simulink model "simulateur_derniere_version"  (R2022b)
settings: Solver=ode4  StartTime=0.0  StopTime=10  FixedStep=dt  RelTol=1e-3
model workspace: external: MATLAB File /Users/antoine/Desktop/GPH/H2023/Design_2/simulation_équipe_1/init.m (data not in the file)
values from neighbouring files (symbols this model uses):
  distance_corde_capteur = 0.00382    [init.m]
  dt = 0.000125    [init.m]
  f = 110    [init.m]    (also in visualize.m = specs(3,:))
  freq_min = 80    [init.m]
  freq_min_1 = freq_min    (= 80)    [init.m]
  Longueur = 0.44    [init.m]
  mu = 0.010011363636363636    (= 0.0100113636364)    [init.m]
  n = 21    [init.m]
libraries: simulink x1, slpidlib x1, dspstat3 x1
settings Model: Creator=antoine  LastModifiedBy=antoine

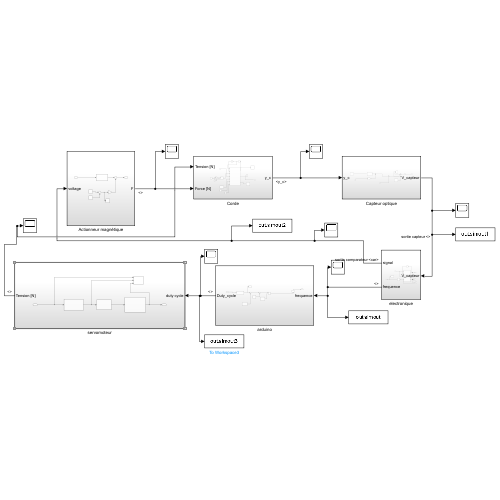
[thumbnail: Simulink's stored preview of the top-level diagram]
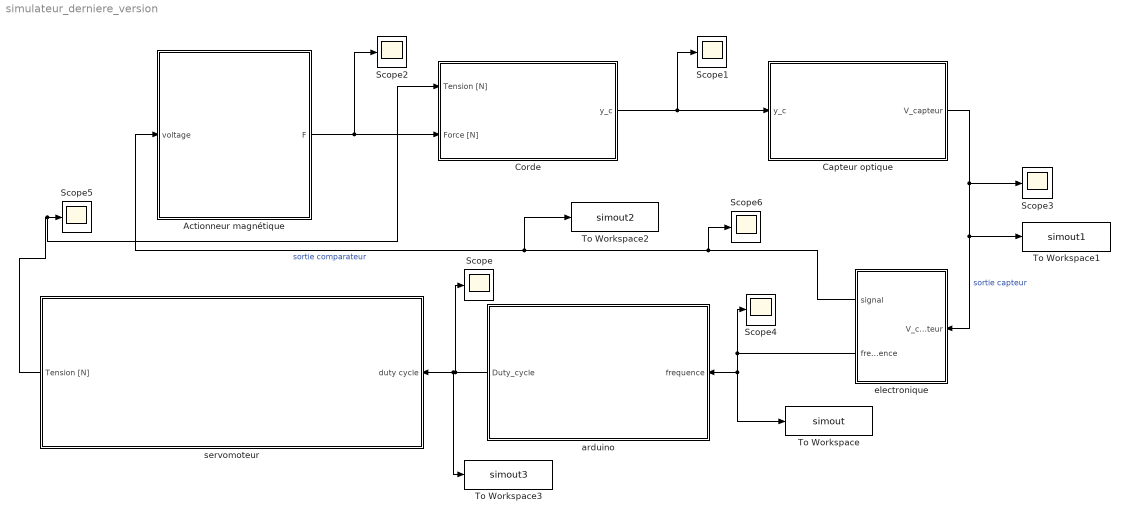
== system simulateur_derniere_version ==
  Actionneur magnétique : Subsystem
  Capteur optique : Subsystem
  Corde : Subsystem
  Scope{,1..6} (7 alike) : Scope
  To Workspace : ToWorkspace  VariableName=simout  SaveFormat=Structure  SampleTime=-1
      settings: Save2DSignal=2-D array (concatenate along first dimension)
  To Workspace1 : ToWorkspace  VariableName=simout1  SampleTime=-1
      settings: Save2DSignal=2-D array (concatenate along first dimension)
  To Workspace2 : ToWorkspace  VariableName=simout2  SampleTime=-1
      settings: Save2DSignal=2-D array (concatenate along first dimension)
  To Workspace3 : ToWorkspace  VariableName=simout3  SampleTime=-1
      settings: Save2DSignal=2-D array (concatenate along first dimension)
  arduino : Subsystem
  electronique : Subsystem
  servomoteur : Subsystem
  wires:
  Corde/1(y_c) -> Capteur optique/1(y_c), Scope1/1
  Capteur optique/1(V_capteur) -> Scope3/1, electronique/1(V_capteur), To Workspace1/1  "sortie capteur"
  servomoteur/1(Tension [N]) -> Corde/1(Tension [N]), Scope5/1
  Actionneur magnétique/1(F) -> Scope2/1, Corde/2(Force [N])
  electronique/1(signal) -> Scope6/1, To Workspace2/1, Actionneur magnétique/1(voltage)  "sortie comparateur"
  electronique/2(frequence) -> To Workspace/1, arduino/1(frequence), Scope4/1
  arduino/1(Duty_cycle) -> Scope/1, To Workspace3/1, servomoteur/1(duty cycle)

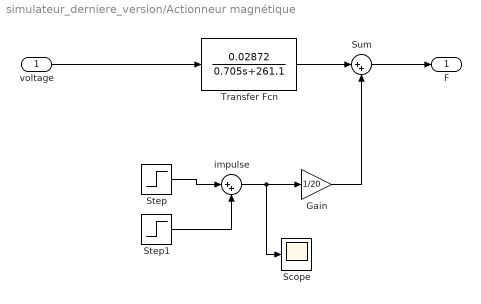
== system simulateur_derniere_version/Actionneur magnétique ==
  voltage : Inport
  Gain : Gain  Gain=1/20
  Scope : Scope
  Step : Step  Time=3*dt  SampleTime=0
  Step1 : Step  Time=6*dt  After=-1  SampleTime=0
  Sum : Sum  Inputs=|++
  Transfer Fcn : TransferFcn  Numerator=[0.02872]  Denominator=[0.705 261.1]
  impulse : Sum  Inputs=|++
  F : Outport
  wires:
  voltage/1 -> Transfer Fcn/1
  Transfer Fcn/1 -> Sum/1
  Sum/1 -> F/1
  Gain/1 -> Sum/2
  Step/1 -> impulse/1
  Step1/1 -> impulse/2
  impulse/1 -> Scope/1, Gain/1

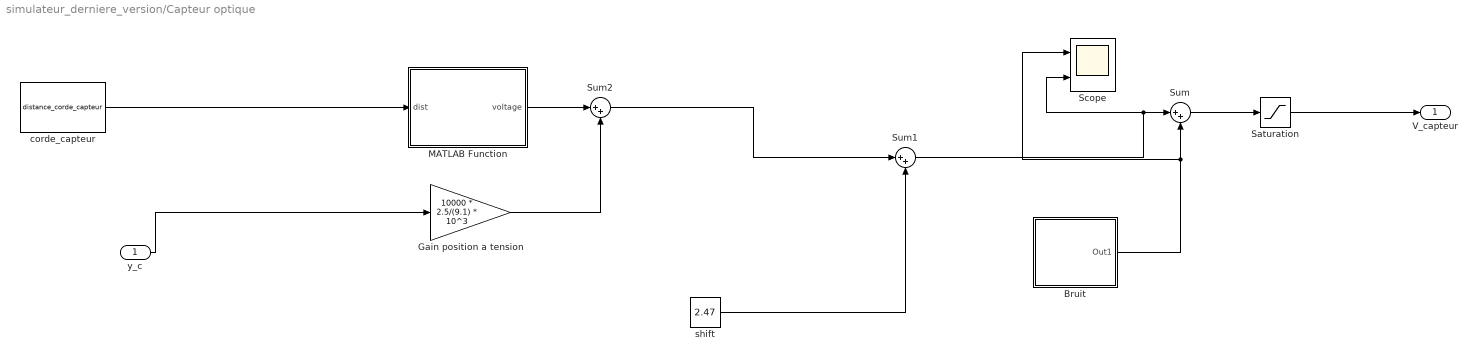
== system simulateur_derniere_version/Capteur optique ==
  y_c : Inport
  Bruit : Subsystem
  Gain position a tension : Gain  Gain=10000 * 2.5/(9.1) * 10^3
  MATLAB Function : MATLAB Function  TreatAsAtomicUnit=on
  Saturation : Saturate  UpperLimit=5  LowerLimit=0
  Scope : Scope  NumInputPorts=2
  Sum : Sum  Inputs=|++
  Sum1 : Sum  Inputs=|++
  Sum2 : Sum  Inputs=|++
  corde_capteur : Constant  Value=distance_corde_capteur
  shift : Constant  Value=2.47
  V_capteur : Outport
  wires:
  Sum/1 -> Saturation/1
  shift/1 -> Sum1/2
  Sum1/1 -> Scope/2, Sum/1
  Bruit/1(Out1) -> Scope/1, Sum/2
  Saturation/1 -> V_capteur/1
  y_c/1 -> Gain position a tension/1
  corde_capteur/1 -> MATLAB Function/1(dist)
  Gain position a tension/1 -> Sum2/2
  Sum2/1 -> Sum1/1
  MATLAB Function/1(voltage) -> Sum2/1

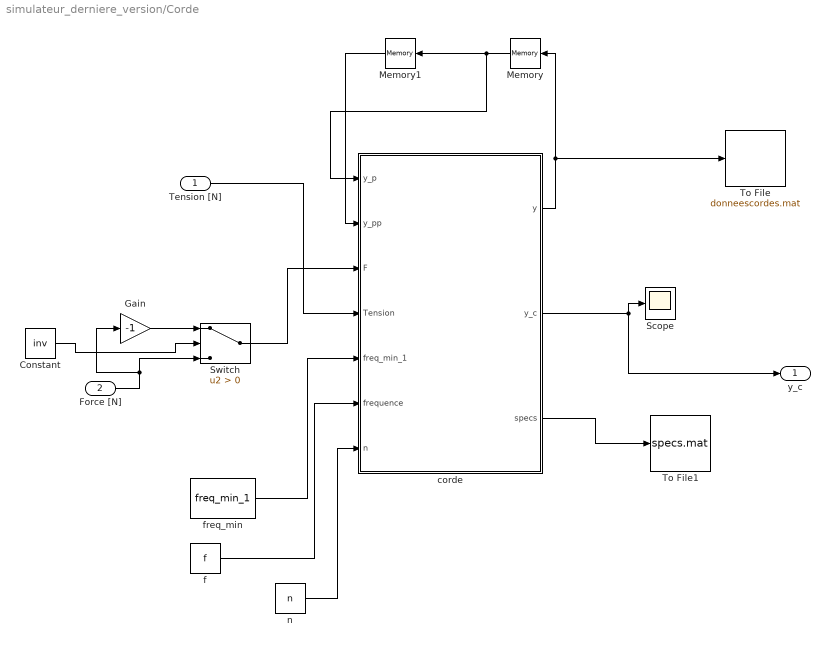
== system simulateur_derniere_version/Corde ==
  Tension [N] : Inport
  Force [N] : Inport  Port=2
  Constant : Constant  Value=inv
  Gain : Gain  Gain=-1
  Memory : Memory
  Memory1 : Memory
  Scope : Scope
  Switch : Switch  Criteria=u2 > Threshold  SaturateOnIntegerOverflow=off  InputSameDT=off
  To File : ToFile  Filename=donneescordes.mat  SaveFormat=Timeseries
  To File1 : ToFile  Filename=specs.mat  MatrixName=specs
  corde : MATLAB Function  TreatAsAtomicUnit=on
  f : Constant  Value=f
  freq_min : Constant  Value=freq_min_1
  n : Constant  Value=n
  y_c : Outport
  wires:
  corde/2(y_c) -> y_c/1, Scope/1
  Memory/1 -> corde/1(y_p), Memory1/1
  Memory1/1 -> corde/2(y_pp)
  corde/1(y) -> Memory/1, To File/1
  Switch/1 -> corde/3(F)
  Gain/1 -> Switch/1
  Force [N]/1 -> Switch/3, Gain/1
  Constant/1 -> Switch/2
  Tension [N]/1 -> corde/4(Tension)
  corde/3(specs) -> To File1/1
  freq_min/1 -> corde/5(freq_min_1)
  f/1 -> corde/6(frequence)
  n/1 -> corde/7(n)

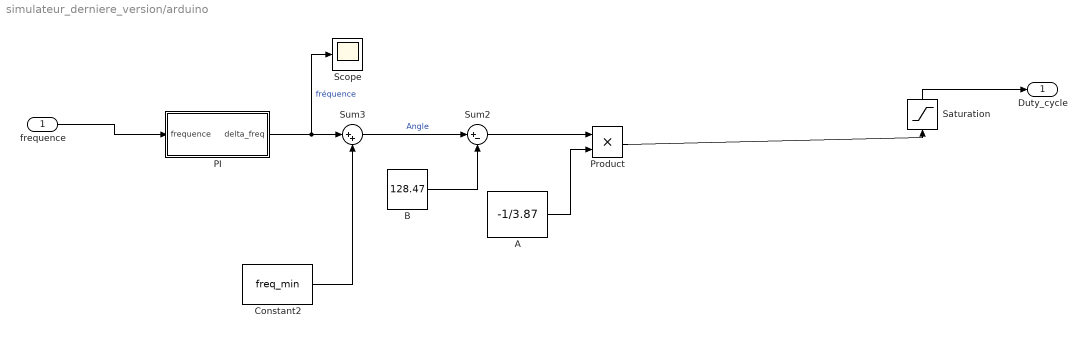
== system simulateur_derniere_version/arduino ==
  frequence : Inport
  A : Constant  Value=-1/3.87
  B : Constant  Value=128.47
  Constant2 : Constant  Value=freq_min
  PI : Subsystem
  Product : Product
  Saturation : Saturate  UpperLimit=11.79  LowerLimit=2.72
  Scope : Scope
  Sum2 : Sum  Inputs=|+-
  Sum3 : Sum  Inputs=|++
  Duty_cycle : Outport
  wires:
  PI/1(delta_freq) -> Sum3/1, Scope/1  "fréquence"
  frequence/1 -> PI/1(frequence)
  Saturation/1 -> Duty_cycle/1
  B/1 -> Sum2/2
  Sum2/1 -> Product/1
  A/1 -> Product/2
  Product/1 -> Saturation/1
  Sum3/1 -> Sum2/1  "Angle"
  Constant2/1 -> Sum3/2

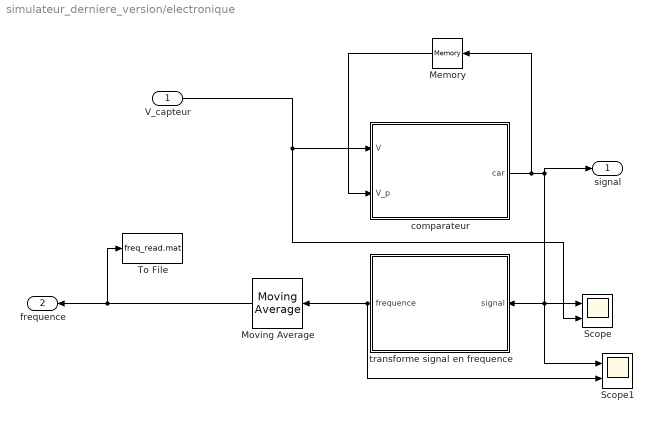
== system simulateur_derniere_version/electronique ==
  V_capteur : Inport
  Memory : Memory
  Moving Average : dspstat3/Moving Average  Method=Sliding window  ForgettingFactorPort=off  SpecifyWindowLength=on  WindowLength=100  OverlapLength=99  AllowArbitraryInputLength=off  ForgettingFactor=0.99  SimulateUsing=Interpreted execution
  Scope : Scope  NumInputPorts=2
  Scope1 : Scope  NumInputPorts=2
  To File : ToFile  Filename=freq_read.mat  MatrixName=freq
  comparateur : MATLAB Function  TreatAsAtomicUnit=on
  transforme signal en frequence : Subsystem
  signal : Outport
  frequence : Outport  Port=2
  wires:
  comparateur/1(car) -> Scope1/1, transforme signal en frequence/1(signal), Scope/1, signal/1, Memory/1
  Memory/1 -> comparateur/2(V_p)
  V_capteur/1 -> Scope/2, comparateur/1(V)
  transforme signal en frequence/1(frequence) -> Scope1/2, Moving Average/1
  Moving Average/1 -> To File/1, frequence/1

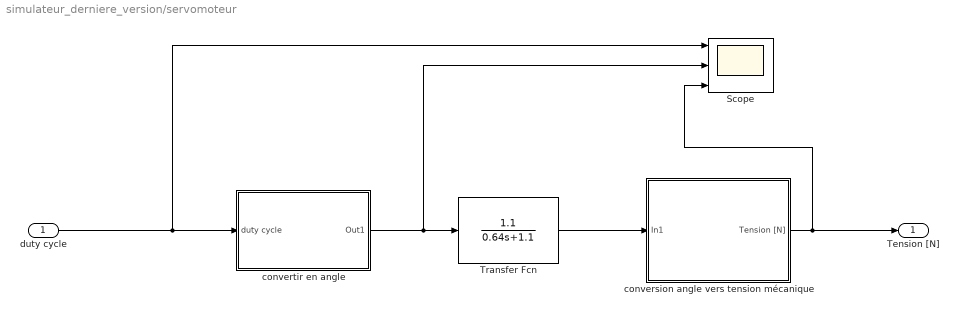
== system simulateur_derniere_version/servomoteur ==
  duty cycle : Inport
  Scope : Scope  NumInputPorts=3
  Transfer Fcn : TransferFcn  Numerator=[1.1]  Denominator=[0.64 1.1]
  conversion angle vers tension mécanique : Subsystem
  convertir en angle : Subsystem
  Tension [N] : Outport
  wires:
  convertir en angle/1(Out1) -> Transfer Fcn/1, Scope/2
  conversion angle vers tension mécanique/1(Tension [N]) -> Scope/3, Tension [N]/1
  duty cycle/1 -> Scope/1, convertir en angle/1(duty cycle)
  Transfer Fcn/1 -> conversion angle vers tension mécanique/1(In1)

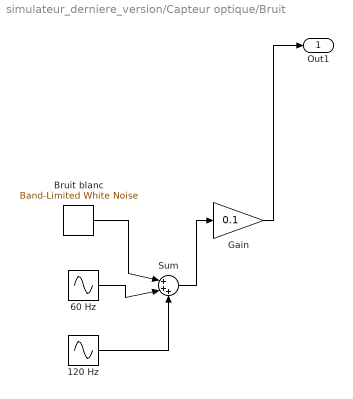
== system simulateur_derniere_version/Capteur optique/Bruit ==
  120 Hz : Sin  Frequency=120  SampleTime=0
  60 Hz : Sin  Frequency=60  SampleTime=0
  Bruit blanc : simulink/Sources/Band-Limited White Noise  Cov=[0.1]  Ts=0.1  seed=[23341]
  Gain : Gain  Gain=0.1
  Sum : Sum  Inputs=|+++
  Out1 : Outport
  wires:
  Bruit blanc/1 -> Sum/1
  60 Hz/1 -> Sum/2
  120 Hz/1 -> Sum/3
  Sum/1 -> Gain/1
  Gain/1 -> Out1/1

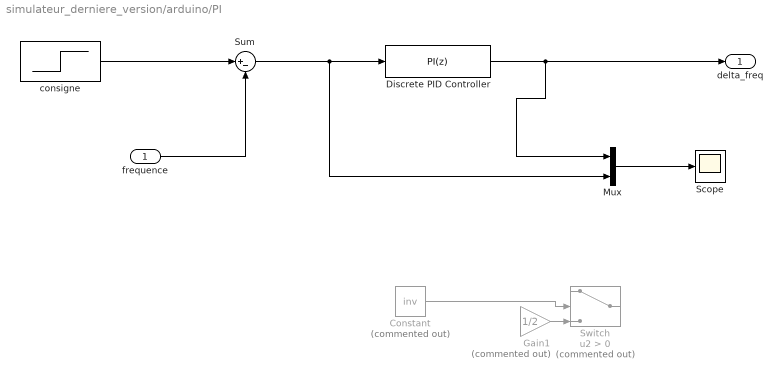
== system simulateur_derniere_version/arduino/PI ==
  frequence : Inport
  Constant : Constant  Commented=on  Value=inv
  Discrete PID Controller : slpidlib/PID Controller  Controller=PI  Form=Ideal  TimeDomain=Discrete-time  UseExternalTs=off  SampleTime=-1  IntegratorMethod=Trapezoidal  FilterMethod=Trapezoidal  ControllerParametersSource=internal  P=-0.5  I=4.1  UseKiTs=off  D=0.4  N=10  UseFilter=on  TunerSelectOption=Transfer Function Based (PID Tuner App)  InitialConditionSource=internal  InitialConditionForIntegrator=0  InitialConditionForFilter=0  DifferentiatorICPrevScaledInput=0  ExternalReset=none  TrackingMode=off  Kt=1  LimitOutput=on  SatLimitsSource=internal  UpperSaturationLimit=1000  LowerSaturationLimit=-1000  LinearizeAsGain=off  AntiWindupMode=clamping  Kb=1  LimitIntegrator=on  UpperIntegratorSaturationLimit=1000  LowerIntegratorSaturationLimit=-1000  POutMin=[-1000]  POutMax=[1000]  IOutMin=[-1000]  IOutMax=[1000]  DOutMin=[-1000]  DOutMax=[1000]  NOutMin=[-1000]  NOutMax=[1000]  SumOutMin=[-1000]  SumOutMax=[1000]  SaturationOutMin=[]  SaturationOutMax=[]  PParamMin=[]  PParamMax=[]  IParamMin=[]  IParamMax=[]  DParamMin=[]  DParamMax=[]  NParamMin=[]  NParamMax=[]  KbParamMin=[]  KbParamMax=[]  KtParamMin=[]  KtParamMax=[]  KbOutMin=[]  KbOutMax=[]  KtOutMin=[]  KtOutMax=[]  IntegratorOutMin=[]  IntegratorOutMax=[]  FilterOutMin=[]  FilterOutMax=[]  SumI1OutMin=[]  SumI1OutMax=[]  SumI2OutMin=[]  SumI2OutMax=[]  SumI3OutMin=[]  SumI3OutMax=[]  SumI4OutMin=[]  SumI4OutMax=[]  SumDOutMin=[]  SumDOutMax=[]  DifferentiatorOutMin=[]  DifferentiatorOutMax=[]  FilterDiffOutCoefMin=[]  FilterDiffOutCoefMax=[]  ReciprocalOutMin=[]  ReciprocalOutMax=[]  SumDenOutMin=[]  SumDenOutMax=[]  SumNumOutMin=[]  SumNumOutMax=[]  DivideOutMin=[]  DivideOutMax=[]  UdiffTsProdOutMin=[]  UdiffTsProdOutMax=[]  NTsProdOutMin=[]  NTsProdOutMax=[]  UintegralTsProdOutMin=[]  UintegralTsProdOutMax=[]  UngainTsProdOutMin=[]  UngainTsProdOutMax=[]  ClampingZeroOutDataTypeStr=Inherit: Inherit via back propagation  ClampingZeroOutMin=[]  ClampingZeroOutMax=[]  FilterDenConstantOutDataTypeStr=Inherit: Inherit via back propagation  FilterDenConstantOutMin=[]  FilterDenConstantOutMax=[]  PCopyOutDataTypeStr=Inherit: Inherit via back propagation  PCopyOutMin=[]  PCopyOutMax=[]  NCopyOutDataTypeStr=Inherit: Inherit via back propagation  NCopyOutMin=[]  NCopyOutMax=[]  IntegratorContinuousStateAttributes=''  IntegratorStateMustResolveToSignalObject=off  IntegratorRTWStateStorageClass=Auto  FilterContinuousStateAttributes=''  FilterStateMustResolveToSignalObject=off  FilterRTWStateStorageClass=Auto  ParallelPVariant=Passthrough  IdealPVariant=InternalParameters  IVariant=InternalParameters  DVariant=Disabled  IntegratorVariant=Discrete  SatVariant=Enabled  AWVariant=DiscClampingIdeal  PCopyVariant=InternalParamsIdeal  TRVariant=Disabled  FdbkBlocksVariant=Feedback  IdealPFdbkVariant=InternalParameters  SatFdbkVariant=Passthrough  DerivativeFilterVariant=Disabled  NVariant=Disabled  NCopyVariant=Disabled_SignalSpec  FilterICVariant=Disabled  IntegratorICVariant=InternalICs  ExternalResetVariant=Disabled  TRSumVariant=Passthrough  SumFdbkVariant=Enabled  SumVariant=Sum_PI  TsampFilterVariant=InternalTs  TsampNgainVariant=Passthrough  TsampIntegralVariant=Passthrough  ExternalSaturationOutDataTypeStr=Inherit: Same as second input
      settings: LibrarySourceBlock=simulink/Discrete/Discrete PID Controller
  Gain1 : Gain  Commented=on  Gain=1/2
  Mux : Mux  Inputs=2
  Scope : Scope
  Sum : Sum  Inputs=|+-
  Switch : Switch  Commented=on  Criteria=u2 > Threshold  SaturateOnIntegerOverflow=off  InputSameDT=off
  consigne : Step  Time=0  After=f  SampleTime=10
  delta_freq : Outport
  wires:
  Mux/1 -> Scope/1
  consigne/1 -> Sum/1
  Sum/1 -> Discrete PID Controller/1, Mux/2
  Discrete PID Controller/1 -> delta_freq/1, Mux/1
  Constant/1 -> Switch/2
  Gain1/1 -> Switch/3
  frequence/1 -> Sum/2

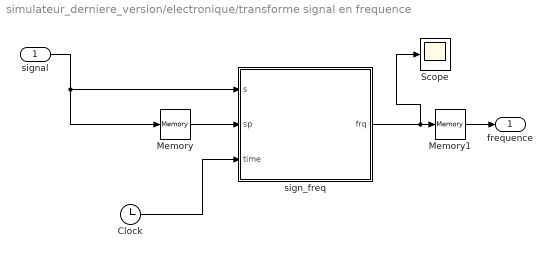
== system simulateur_derniere_version/electronique/transforme signal en frequence ==
  signal : Inport
  Clock : Clock
  Memory : Memory  InitialCondition=5
  Memory1 : Memory  InitialCondition=100
  Scope : Scope
  sign_freq : MATLAB Function  TreatAsAtomicUnit=on
  frequence : Outport
  wires:
  signal/1 -> Memory/1, sign_freq/1(s)
  sign_freq/1(frq) -> Memory1/1, Scope/1
  Clock/1 -> sign_freq/3(time)
  Memory/1 -> sign_freq/2(sp)
  Memory1/1 -> frequence/1

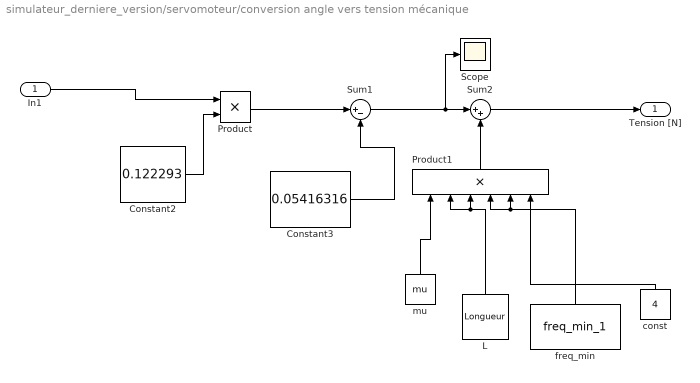
== system simulateur_derniere_version/servomoteur/conversion angle vers tension mécanique ==
  In1 : Inport
  Constant2 : Constant  Value=0.122293
  Constant3 : Constant  Value=0.05416316
  L : Constant  Value=Longueur
  Product : Product
  Product1 : Product  Inputs=6
  Scope : Scope
  Sum1 : Sum  Inputs=|+-
  Sum2 : Sum  Inputs=|++
  const : Constant  Value=4
  freq_min : Constant  Value=freq_min_1
  mu : Constant  Value=mu
  Tension [N] : Outport
  wires:
  Constant2/1 -> Product/2
  In1/1 -> Product/1
  Sum1/1 -> Sum2/1, Scope/1
  Product/1 -> Sum1/1
  Constant3/1 -> Sum1/2
  Sum2/1 -> Tension [N]/1
  Product1/1 -> Sum2/2
  mu/1 -> Product1/1
  L/1 -> Product1/2, Product1/3
  freq_min/1 -> Product1/4, Product1/5
  const/1 -> Product1/6

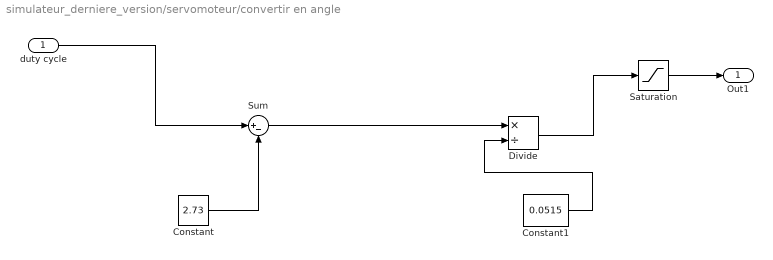
== system simulateur_derniere_version/servomoteur/convertir en angle ==
  duty cycle : Inport
  Constant : Constant  Value=2.73
  Constant1 : Constant  Value=0.0515
  Divide : Product  Inputs=*/
  Saturation : Saturate  UpperLimit=170  LowerLimit=0
  Sum : Sum  Inputs=|+-
  Out1 : Outport
  wires:
  Constant/1 -> Sum/2
  Constant1/1 -> Divide/2
  Sum/1 -> Divide/1
  duty cycle/1 -> Sum/1
  Divide/1 -> Saturation/1
  Saturation/1 -> Out1/1

== matlab function simulateur_derniere_version/Capteur optique/MATLAB Function ==
  data: dist input; voltage output
function voltage = distance_vers_voltage(dist)
    dist_pouce = dist*0.0393701;
    voltage = exp(-120*(dist_pouce-0.17)^2);
end

== matlab function simulateur_derniere_version/Corde/corde ==
  data: y output size=[1, n] [1..1000]; y_p input size=[1, n]; y_pp input size=[1, n]; y_c output size=1; F input size=1; Tension input; freq_min_1 input; frequence input; specs output; n input
function [y,y_c,specs] = corde(y_p, y_pp,F, Tension,freq_min_1,frequence,n)

dt = 0.000125;
beta = 3.2 * 10^(-3);
mu = 7.68 * 10^(-3); % [kg/m]
masse = 0.004405; % [kg s]
Longueur = 0.44; % [m]
%mu = masse/Longueur; % 
%freq_min = 40;

T_init = freq_min_1^2 * 4 * Longueur^2 * mu;

%if time < 0.03
%    T = T_init;  % f^2 * 4 * Longueur^2 * mu;%/mode^2; %f_1^2 * 4 * Longueur^2 * mu;
%else
%    T = Tension;
%end
T = Tension;
n = 21; % découper la corde en 'n' morceaux

p_actionneur = 16;
p_capteur = 5;

dx = Longueur/(n-1);

%c = sqrt(T/(mu));


y = zeros(1,n);
f = zeros(1,n);
f(p_actionneur) = F;

for i = 2:(n - 1)
    pos = (y_p(i+1)-2*y_p(i)+y_p(i-1));
    first = (dt^2)/(mu + beta*dt);
    y(i) = first*(T*pos/dx^2 + mu*(2*y_p(i) - y_pp(i))/(dt^2) +beta*y_p(i)/dt +f(i));
end
y_c = y(p_capteur);
specs = [T frequence];

% Calcul constante de la simulation


end

== matlab function simulateur_derniere_version/electronique/comparateur ==
  data: V input; car output; V_p input
function car = comparateur(V, V_p)

if V <= 2
    car = 0;
elseif V >= 3
    car = 5;
else
    car = V_p;
end
end

== matlab function simulateur_derniere_version/electronique/transforme signal en frequence/sign_freq ==
  settings: updateMethod=DISCRETE
  data: s input; sp input; frq output; time input
function frq = sign_freq(s, sp, time)
persistent up_timer;
persistent down_timer;
% section pour pas avoir de bug
if isempty(up_timer)
    up_timer = 0;
end
if isempty(down_timer)
    down_timer = 0;
    frq = 100;
end
% pas de bug



if s == 5 && sp ~= 5 % debut du up
    up_timer = time;
elseif s == 0 && sp ~= 0 % debut du down
    down_timer = time;
end
period = abs((up_timer-down_timer)*2);
frq = 1/period;
